simulink model "lin_2DoF"  (R2025a)
settings: Solver=VariableStepAuto  StartTime=0.0  StopTime=150  RelTol=1e-3
settings Model: Creator=jidki  LastModifiedBy=jidki

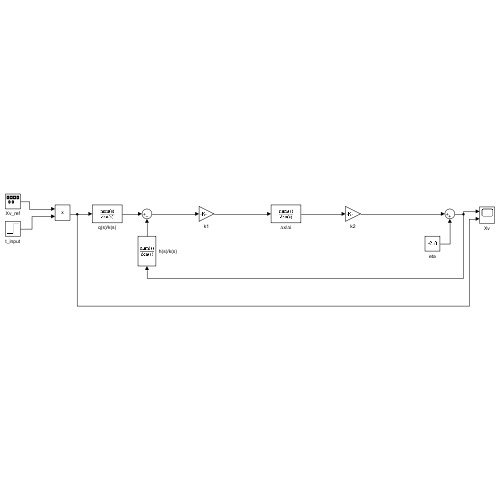
[thumbnail: Simulink's stored preview of the top-level diagram]
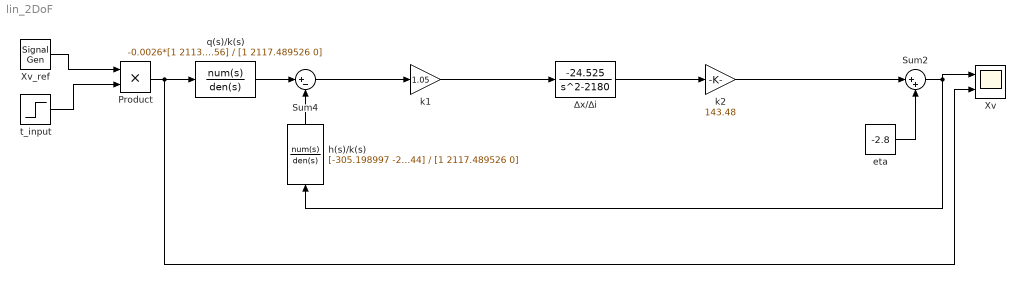
== system lin_2DoF ==
  Product : Product
  Sum2 : Sum  Inputs=|++
  Sum4 : Sum  Inputs=|+-
  Xv : Scope  NumInputPorts=2
      settings: ActiveDisplayYMinimum=-3.3692507773662936  ActiveDisplayYMaximum=2.3232569962966436
  Xv_ref : SignalGenerator  WaveForm=square  Amplitude=143.48*0.009  Frequency=1/5  Units=rad/sec
  eta : Constant  Value=-2.8
  h(s)/k(s) : TransferFcn  Numerator=[-305.198997 -2531.996576 -2834.571544]  Denominator=[1 2117.489526 0]
  k1 : Gain  Gain=1.05
  k2 : Gain  Gain=143.48
  q(s)/k(s) : TransferFcn  Numerator=-0.0026*[1 2113.2 1116403.56]  Denominator=[1 2117.489526 0]
  t_input : Step  Time=25  SampleTime=0
  ∆x/∆i : TransferFcn  Numerator=[-24.525]  Denominator=[1 0 -2180]
  wires:
  eta/1 -> Sum2/2
  k2/1 -> Sum2/1
  k1/1 -> ∆x/∆i/1
  Product/1 -> Xv/2, q(s)/k(s)/1
  ∆x/∆i/1 -> k2/1
  Sum2/1 -> h(s)/k(s)/1, Xv/1
  h(s)/k(s)/1 -> Sum4/2
  q(s)/k(s)/1 -> Sum4/1
  Sum4/1 -> k1/1
  t_input/1 -> Product/2
  Xv_ref/1 -> Product/1
